simulink model "controller_real"  (R2023b)
settings: Solver=FixedStepAuto  StartTime=0.0  StopTime=5  RelTol=1e-3  EnableMultiTasking=on
undefined symbols (not defined in the file): accDirDisc, accInt, C, F, G, k_awp, K_i_disc, K_r_disc, L_disc, T, targetPos
libraries: mbedblockslib x6, simulink x2
settings Model: ExtModeTrigDuration=10  Creator=miqui  LastModifiedBy=miqui
settings OptimizationCC: EnhancedBackFolding=on  PassReuseOutputArgsAs=Individual arguments  ZeroExternalMemoryAtStartup=off  ZeroInternalMemoryAtStartup=off  MaxStackSize=64  OptimizeBlockOrder=speed  DifferentSizesBufferReuse=on  OptimizationCustomize=off  EfficientTunableParamExpr=on
settings DebuggingCC: ParameterTunabilityLossMsg=error
settings HardwareCC: ProdBitPerPointer=32  ProdBitPerSizeT=32  ProdBitPerPtrDiffT=32  ProdLargestAtomicInteger=Long  ProdLargestAtomicFloat=Double  ProdWordSize=32  ProdLongLongMode=on  ProdHWDeviceType=ARM Compatible->ARM Cortex  UseEmbeddedCoderFeatures=off
settings SFSimCC: MATLABDynamicMemAlloc=off
settings RTWCC: Description=Embedded Coder  SystemTargetFile=ert.tlc  HardwareBoard=STM32 Nucleo F411RE  TemplateMakefile=ert_default_tmf  Toolchain=GNU Tools for ARM Embedded Processors
settings CodeAppCC: ForceParamTrailComments=on  IgnoreCustomStorageClasses=off  OperatorAnnotations=on  SimulinkDataObjDesc=on  SFDataObjDesc=on  InsertBlockDesc=on
settings ERTTargetCC: SupportNonInlinedSFcns=on  ExtModeTransport=3  ExtModeStaticAlloc=on  ExtModeStaticAllocSize=2000  ExtModeMexFile=ext_xcp  ExtModeIntrfLevel=Level2 - Open

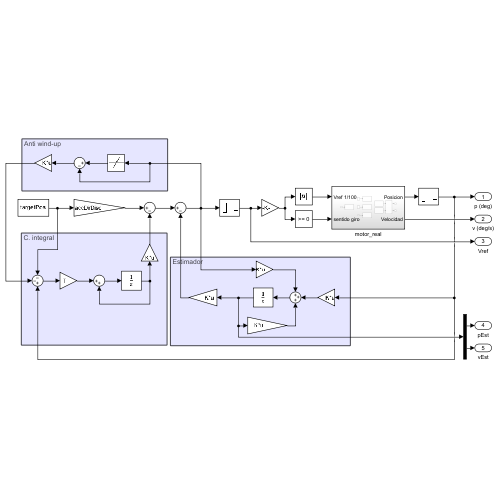
[thumbnail: Simulink's stored preview of the top-level diagram]
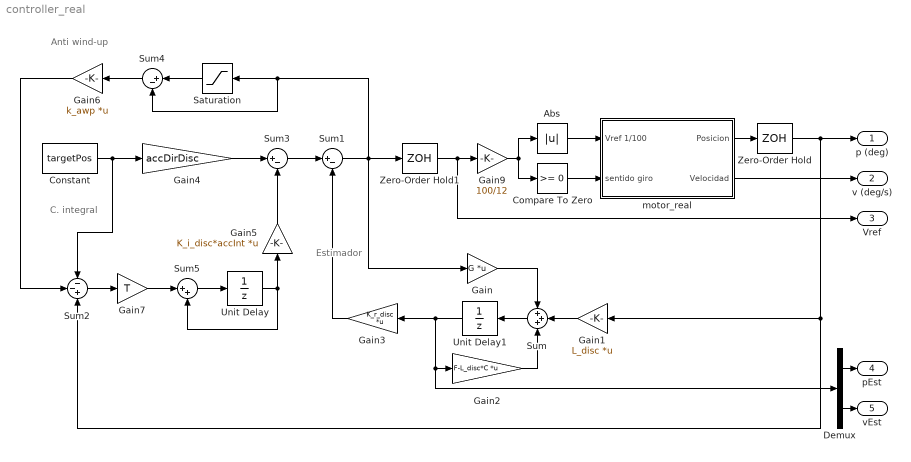
== system controller_real ==
  note: Anti wind-up
  note: Estimador
  note: C. integral
  Abs : Abs  SaturateOnIntegerOverflow=off
  Compare To Zero : simulink/Logic and Bit Operations/Compare To Zero  relop=>=  OutDataTypeStr=boolean
  Constant : Constant  Value=targetPos
  Demux : Demux  Outputs=2
  Gain : Gain  Gain=G  Multiplication=Matrix(K*u)
  Gain1 : Gain  Gain=L_disc  Multiplication=Matrix(K*u)
  Gain2 : Gain  Gain=F-L_disc*C  Multiplication=Matrix(K*u)
  Gain3 : Gain  Gain=K_r_disc  Multiplication=Matrix(K*u)
  Gain4 : Gain  Gain=accDirDisc
  Gain5 : Gain  Gain=K_i_disc*accInt  Multiplication=Matrix(K*u)
  Gain6 : Gain  Gain=k_awp  Multiplication=Matrix(K*u)
  Gain7 : Gain  Gain=T
  Gain9 : Gain  Gain=100/12
  Saturation : Saturate  UpperLimit=12  LowerLimit=-12
  Sum : Sum  Inputs=+++
  Sum1 : Sum  Inputs=|+-
  Sum2 : Sum  Inputs=--+
  Sum3 : Sum  Inputs=|+-
  Sum4 : Sum  Inputs=|+-
  Sum5 : Sum  Inputs=|++
  Unit Delay : UnitDelay  SampleTime=T  HasFrameUpgradeWarning=on
  Unit Delay1 : UnitDelay  SampleTime=T  HasFrameUpgradeWarning=on
  Zero-Order Hold : ZeroOrderHold  SampleTime=T
  Zero-Order Hold1 : ZeroOrderHold  SampleTime=T
  motor_real : Subsystem
  p (deg) : Outport
  v (deg/s) : Outport  Port=2
  Vref : Outport  Port=3
  pEst : Outport  Port=4
  vEst : Outport  Port=5
  wires:
  Zero-Order Hold/1 -> p (deg)/1, Gain1/1, Sum2/3
  Sum3/1 -> Sum1/1
  Unit Delay/1 -> Sum5/2, Gain5/1
  Gain7/1 -> Sum5/1
  Sum5/1 -> Unit Delay/1
  Sum1/1 -> Saturation/1, Sum4/2, Zero-Order Hold1/1, Gain/1
  Zero-Order Hold1/1 -> Gain9/1, Vref/1
  Demux/1 -> pEst/1
  Gain1/1 -> Sum/2
  Gain5/1 -> Sum3/2
  Gain6/1 -> Sum2/2
  Demux/2 -> vEst/1
  Constant/1 -> Gain4/1, Sum2/1
  Gain4/1 -> Sum3/1
  Unit Delay1/1 -> Demux/1, Gain2/1, Gain3/1
  Sum4/1 -> Gain6/1
  Sum2/1 -> Gain7/1
  Gain2/1 -> Sum/3
  Gain/1 -> Sum/1
  Saturation/1 -> Sum4/1
  Sum/1 -> Unit Delay1/1
  Gain3/1 -> Sum1/2
  motor_real/1(Posicion) -> Zero-Order Hold/1
  motor_real/2(Velocidad) -> v (deg/s)/1
  Abs/1 -> motor_real/1(Vref 1/100)
  Compare To Zero/1 -> motor_real/2(sentido giro)
  Gain9/1 -> Abs/1, Compare To Zero/1

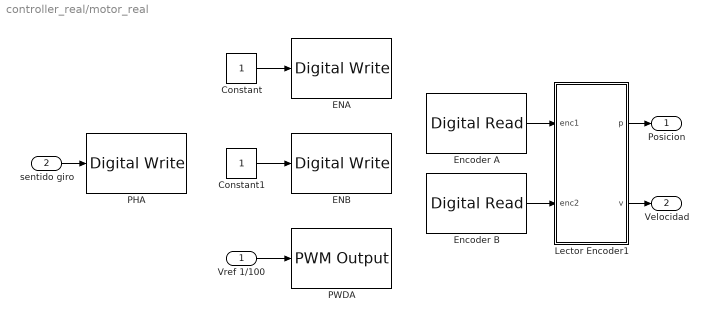
== system controller_real/motor_real ==
  Vref 1/100 : Inport
  sentido giro : Inport  Port=2
  Constant : Constant
  Constant1 : Constant
  ENA : mbedblockslib/Digital Write  Pin=D2  Direction=output
      settings: LibrarySourceBlock=stmnucleorootlib/Common/Digital Write
  ENB : mbedblockslib/Digital Write  Pin=D11  Direction=output
      settings: LibrarySourceBlock=stmnucleorootlib/Common/Digital Write
  Encoder A : mbedblockslib/Digital Read  Pin=A1  Direction=input  SampleTime=0.0001
      settings: LibrarySourceBlock=stmnucleorootlib/Common/Digital Read
  Encoder B : mbedblockslib/Digital Read  Pin=A0  Direction=input  SampleTime=0.0001
      settings: LibrarySourceBlock=stmnucleorootlib/Common/Digital Read
  Lector Encoder1 : Subsystem
  PHA : mbedblockslib/Digital Write  Pin=D3  Direction=output
      settings: LibrarySourceBlock=stmnucleorootlib/Common/Digital Write
  PWDA : mbedblockslib/PWM Output  Pin=D5  EnableInputFrequency=off  InitialFrequency=5000  InitialDutyCycle=0  NotificationType=None
      settings: LibrarySourceBlock=stmnucleorootlib/Common/PWM Output
  Posicion : Outport
  Velocidad : Outport  Port=2
  wires:
  sentido giro/1 -> PHA/1
  Constant/1 -> ENA/1
  Constant1/1 -> ENB/1
  Vref 1/100/1 -> PWDA/1
  Encoder A/1 -> Lector Encoder1/1(enc1)
  Encoder B/1 -> Lector Encoder1/2(enc2)
  Lector Encoder1/2(v) -> Velocidad/1
  Lector Encoder1/1(p) -> Posicion/1

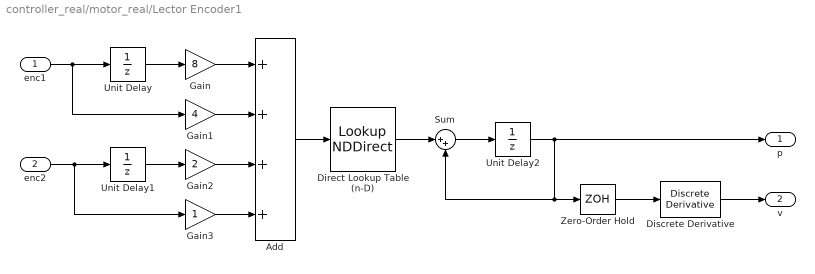
== system controller_real/motor_real/Lector Encoder1 ==
  enc1 : Inport
  enc2 : Inport  Port=2
  Add : Sum  Inputs=++++  OutDataTypeStr=double
  Direct Lookup Table (n-D) : LookupNDDirect  NumberOfTableDimensions=1  Table=[0,-1,1,0,1,0,0,-1,-1,0,0,1,0,1,-1,0]
  Discrete Derivative : simulink/Discrete/Discrete Derivative  gainval=1.0  ICPrevScaledInput=0.0  OutMin=[]  OutMax=[]  OutDataType=fixdt(1, 16)  OutScaling=2^-10  DoSatur=off
  Gain : Gain  Gain=8
  Gain1 : Gain  Gain=4
  Gain2 : Gain  Gain=2
  Gain3 : Gain
  Sum : Sum  Inputs=|++
  Unit Delay : UnitDelay  SampleTime=-1  HasFrameUpgradeWarning=on
  Unit Delay1 : UnitDelay  SampleTime=-1  HasFrameUpgradeWarning=on
  Unit Delay2 : UnitDelay  SampleTime=-1  HasFrameUpgradeWarning=on
  Zero-Order Hold : ZeroOrderHold  SampleTime=0.01
  p : Outport
  v : Outport  Port=2
  wires:
  enc1/1 -> Unit Delay/1, Gain1/1
  enc2/1 -> Unit Delay1/1, Gain3/1
  Unit Delay/1 -> Gain/1
  Unit Delay1/1 -> Gain2/1
  Gain/1 -> Add/1
  Gain1/1 -> Add/2
  Gain2/1 -> Add/3
  Gain3/1 -> Add/4
  Add/1 -> Direct Lookup Table (n-D)/1
  Direct Lookup Table (n-D)/1 -> Sum/1
  Sum/1 -> Unit Delay2/1
  Unit Delay2/1 -> Zero-Order Hold/1, Sum/2, p/1
  Zero-Order Hold/1 -> Discrete Derivative/1
  Discrete Derivative/1 -> v/1
